simulink model "exp06"  (R2021a)
settings: Solver=VariableStepAuto  StartTime=0.0  StopTime=5.00  RelTol=1e-3
libraries: spsIGBTDiodeLib x8, spsDCVoltageSourceLib x2, spsSeriesRLCBranchLib x1, spsTriangleGeneratorLib x1, spsVoltageMeasurementLib x1, spspowerguiLib x1
settings Model: Creator=User  LastModifiedBy=User

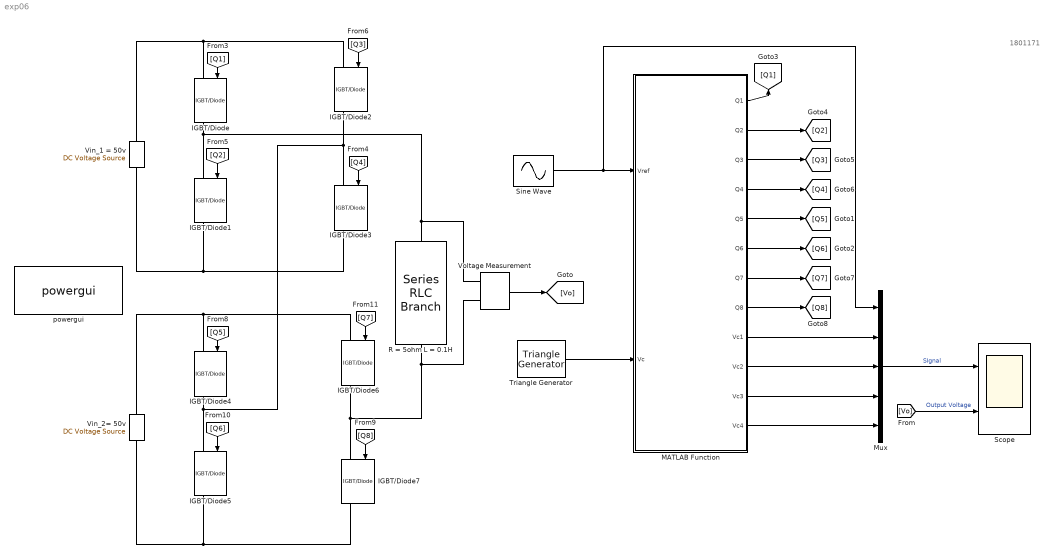
== system exp06 ==
  note: 1801171
  IGBT/Diode{,1..7} (8 alike) : spsIGBTDiodeLib/IGBT//Diode  Ron=1e-3  Rs=1e5  Cs=inf  Measurements=on
  MATLAB Function : MATLAB Function  TreatAsAtomicUnit=on
  Mux : Mux  Inputs=5
  R = 5ohm L = 0.1H : spsSeriesRLCBranchLib/Series RLC Branch  LConnTagsString=__new0  RConnTagsString=__new0  BranchType=RL  Resistance=5  Inductance=100e-3  SetiL0=off  InitialCurrent=0  Capacitance=1e-6  Setx0=off  InitialVoltage=0  Measurements=None
  Scope : Scope  NumInputPorts=2
  Sine Wave : Sin  Frequency=2*pi*50  SampleTime=0
  Triangle Generator : spsTriangleGeneratorLib/Triangle Generator  Freq=1000  Phase=0  Ts=0
  Vin_1 = 50v : spsDCVoltageSourceLib/DC Voltage Source  Amplitude=50  Measurements=None
  Vin_2= 50v : spsDCVoltageSourceLib/DC Voltage Source  Amplitude=50  Measurements=None
  Voltage Measurement : spsVoltageMeasurementLib/Voltage Measurement  PhasorSimulation=off  OutputType=Complex  PSBequivalent=0
  powergui : spspowerguiLib/powergui  Priority=1  SimulationMode=Discrete  SampleTime=0.5e-6  frequency=60  Iterations=50  frequencyindice=0  Pbase=100e6  ErrMax=1e-4  UnitsV=kV  UnitsW=MW  buscounter=0  FunctionMessages=off  echomessages=off  EnableUseOfTLC=off  CurrentSourceSwitches=off  DisableSnubberDevices=off  DisableRonSwitches=off  DisableVfSwitches=off  DisplayEquations=off  AutomaticDiscreteSolvers=off  SolverType=Tustin/Backward Euler (TBE)  Interpol=off  ExternalGateDelay=off  methode=off  Ts=100  x0status=blocks  SPID=on  SwTol=0  HookPort=off  NonlinearTolerance=1e-4  nMaxIteration=100  ContinueOnMaxIteration=off  RestoreLinks=warning  ResistiveCurrentMeasurement=off  Frange=[0:2:500]  Ylog=off  Xlog=on  ShowGrid=off  save=off  variable=ZData  structure=0  ZoomFFT=off  StartTime=0.0  cycles=1  DisplayStyle=1  fundamental=60  FreqAxis=off  MaxFrequency=1000  frequencyindicesteady=1  RmsSteady=1  display=off
  wires:
  Triangle Generator/1 -> MATLAB Function/2(Vc)
  Sine Wave/1 -> Mux/1, MATLAB Function/1(Vref)
  MATLAB Function/3(Q3) -> [Q3]
  [Vo] -> Scope/2  "Output Voltage"
  MATLAB Function/2(Q2) -> [Q2]
  [Q3] -> IGBT/Diode2/1
  [Q4] -> IGBT/Diode3/1
  [Q2] -> IGBT/Diode1/1
  MATLAB Function/4(Q4) -> [Q4]
  Mux/1 -> Scope/1  "SIgnal"
  MATLAB Function/1(Q1) -> [Q1]
  [Q1] -> IGBT/Diode/1
  [Q5] -> IGBT/Diode4/1
  [Q7] -> IGBT/Diode6/1
  [Q8] -> IGBT/Diode7/1
  [Q6] -> IGBT/Diode5/1
  Voltage Measurement/1 -> [Vo]
  MATLAB Function/5(Q5) -> [Q5]
  MATLAB Function/6(Q6) -> [Q6]
  MATLAB Function/7(Q7) -> [Q7]
  MATLAB Function/8(Q8) -> [Q8]
  MATLAB Function/9(Vc1) -> Mux/2
  MATLAB Function/10(Vc2) -> Mux/3
  MATLAB Function/11(Vc3) -> Mux/4
  MATLAB Function/12(Vc4) -> Mux/5
  connections:
  IGBT/Diode2/RConn1 -- IGBT/Diode5/LConn1 -- IGBT/Diode4/RConn1 -- IGBT/Diode3/LConn1
  Vin_1 = 50v/RConn1 -- IGBT/Diode/LConn1 -- IGBT/Diode2/LConn1
  Vin_1 = 50v/LConn1 -- IGBT/Diode3/RConn1 -- IGBT/Diode1/RConn1
  IGBT/Diode1/LConn1 -- Voltage Measurement/LConn1 -- R = 5ohm L = 0.1H/LConn1 -- IGBT/Diode/RConn1
  Vin_2= 50v/LConn1 -- IGBT/Diode7/RConn1 -- IGBT/Diode5/RConn1
  IGBT/Diode4/LConn1 -- Vin_2= 50v/RConn1 -- IGBT/Diode6/LConn1
  IGBT/Diode6/RConn1 -- R = 5ohm L = 0.1H/RConn1 -- Voltage Measurement/LConn2 -- IGBT/Diode7/LConn1

== matlab function exp06/MATLAB Function ==
  data: Vref input; Q1 output; Vc input; Q2 output; Q3 output; Q4 output; Q5 output; Q6 output; Q7 output; Q8 output; Vc1 output; Vc2 output; Vc3 output; Vc4 output
function [Q1 ,Q2 ,Q3 ,Q4,Q5,Q6,Q7,Q8,Vc1,Vc2,Vc3,Vc4] = pulse(Vref, Vc)
Q1=0; Q2=0; Q3=0; Q4=0; Q5=0; Q6=0; Q7=0; Q8=0;
Vc1 = (Vc+1)*0.25;
Vc2 = (Vc+3)*0.25;
Vc3 = (Vc+1)*(-0.25);
Vc4 = (Vc+3)*(-0.25);
if Vref>=0
    if Vref >= 0 && Vref<=0.5
        if Vref>=Vc1
        Q1=1; Q2=0; Q3=0; Q4=1; Q5=1; Q6=0; Q7=1; Q8=0;
    else
        Q1=0; Q2=1; Q3=1; Q4=1; Q5=1; Q6=0; Q7=1; Q8=0;
    end
    else
    if Vref>=Vc2
        Q1=1; Q2=0; Q3=0; Q4=1; Q5=1; Q6=0; Q7=0; Q8=1;
    else
        Q1=1; Q2=0; Q3=0; Q4=1; Q5=1; Q6=0; Q7=1; Q8=0;
    end
    end
end
if Vref<=0
    if Vref<=0 && Vref>=-0.5
        if Vref<=Vc3
        Q1=0; Q2=1; Q3=1; Q4=0; Q5=0; Q6=1; Q7=0; Q8=1;
    else
        Q1=0; Q2=1; Q3=0; Q4=1; Q5=0; Q6=1; Q7=0; Q8=1;
        end
    else
    if Vref<=Vc4
       Q1=0; Q2=1; Q3=1; Q4=0; Q5=1; Q6=0; Q7=0; Q8=1;
    else
        Q1=0; Q2=1; Q3=1; Q4=0; Q5=1; Q6=0; Q7=0; Q8=1;
    end
    end
end
end
